simulink model "lunar_landing_modified"  (R2016b)
settings: Solver=ode5  StartTime=0.0  StopTime=100  FixedStep=0.01  RelTol=1e-3
undefined symbols (not defined in the file or in its folder): sigbuilder_block
settings Model: Creator=Thomas  LastModifiedBy=Thomas

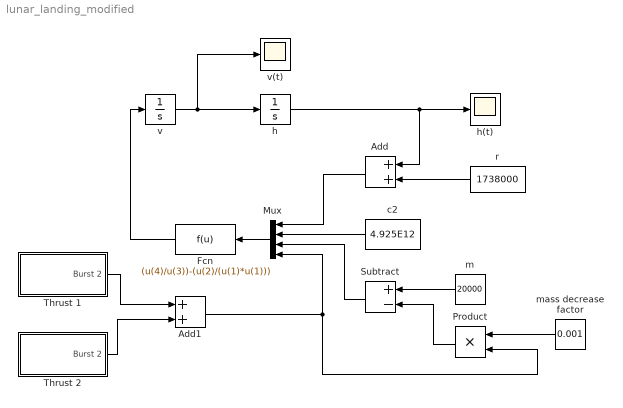
== system lunar_landing_modified ==
  Add : Sum
  Add1 : Sum
  Fcn : Fcn  Expr=(u(4)/u(3))-(u(2)/(u(1)*u(1)))
  Mux : Mux
  Product : Product
  Subtract : Sum  Inputs=+-
  Thrust 1 : Subsystem  Tag=STV Subsys  LoadFcn=sigbuilder_block('load',[448.5 411.75 550.5 334.5 ]);  StartFcn=sigbuilder_block('start');  StopFcn=sigbuilder_block('stop');  ClipboardFcn=sigbuilder_block('clipboard');  mask(Sigbuilder block){tuvar=[0:10]}
      mask help: Simulink:masks:SigbuilderBlock_MD
      mask init:
      | if ~strcmp(get_param(bdroot(gcbh),'SimulationStatus'),'stopped') tuvar = sigbuilder_block('maskInit'); end
      settings: CopyFcn=sigbuilder_block('copy');  DeleteFcn=sigbuilder_block('delete');  ModelCloseFcn=sigbuilder_block('modelClose');  PreSaveFcn=sigbuilder_block('preSave');  PauseFcn=sigbuilder_block('pause');  ContinueFcn=sigbuilder_block('continue');  NameChangeFcn=sigbuilder_block('namechange');  OpenFcn=sigbuilder_block('open',[446.25 33.75 550.5 334.5 ]);  CloseFcn=sigbuilder_block('close');
      mask Display: plot(0, 0, 100, 100,[2, 2, 32, 32, 2], [68, 8, 8, 68, 68],[32, 2], [38, 38], [32, 19, 2],[53, 60, 44], [32, 17, 17, 2],[16, 16, 31, 31]);txt = getActiveGroup(gcbh);text(2, 100, txt,'verticalAlignment', 'top');
  Thrust 2 : Subsystem  Tag=STV Subsys  LoadFcn=sigbuilder_block('load',[450.75 29.25 550.5 334.5 ]);  StartFcn=sigbuilder_block('start');  StopFcn=sigbuilder_block('stop');  ClipboardFcn=sigbuilder_block('clipboard');  mask(Sigbuilder block){tuvar=[0:10]}
      mask help: Simulink:masks:SigbuilderBlock_MD
      mask init:
      | if ~strcmp(get_param(bdroot(gcbh),'SimulationStatus'),'stopped') tuvar = sigbuilder_block('maskInit'); end
      settings: CopyFcn=sigbuilder_block('copy');  DeleteFcn=sigbuilder_block('delete');  ModelCloseFcn=sigbuilder_block('modelClose');  PreSaveFcn=sigbuilder_block('preSave');  PauseFcn=sigbuilder_block('pause');  ContinueFcn=sigbuilder_block('continue');  NameChangeFcn=sigbuilder_block('namechange');  OpenFcn=sigbuilder_block('open',[446.25 33.75 550.5 334.5 ]);  CloseFcn=sigbuilder_block('close');
      mask Display: plot(0, 0, 100, 100,[2, 2, 32, 32, 2], [68, 8, 8, 68, 68],[32, 2], [38, 38], [32, 19, 2],[53, 60, 44], [32, 17, 17, 2],[16, 16, 31, 31]);txt = getActiveGroup(gcbh);text(2, 100, txt,'verticalAlignment', 'top');
  c2 : Constant  Value=4.925E12
  h : Integrator  InitialCondition=1000
  h(t) : Scope
  m : Constant  Value=20000
  mass decrease factor : Constant  Value=0.001
  r : Constant  Value=1738000
  v : Integrator  InitialCondition=-10
  v(t) : Scope
  wires:
  v/1 -> h/1, v(t)/1
  Mux/1 -> Fcn/1
  h/1 -> h(t)/1, Add/1
  r/1 -> Add/2
  Add/1 -> Mux/1
  c2/1 -> Mux/2
  m/1 -> Subtract/1
  Thrust 2/1(Burst 2) -> Add1/2
  Add1/1 -> Product/2, Mux/4
  Fcn/1 -> v/1
  Thrust 1/1(Burst 2) -> Add1/1
  mass decrease factor/1 -> Product/1
  Product/1 -> Subtract/2
  Subtract/1 -> Mux/3

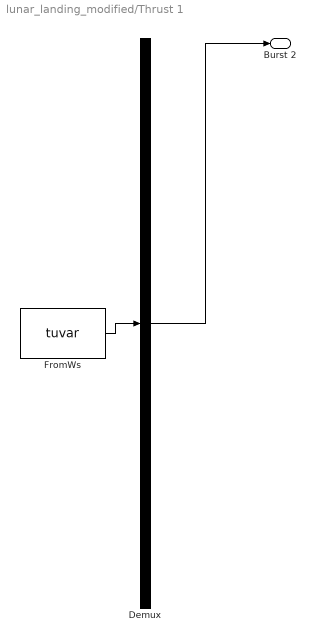
== system lunar_landing_modified/Thrust 1 ==
  Demux : Demux  Tag=STV Demux  Outputs=1
  FromWs : FromWorkspace  Tag=STV FromWs  VariableName=tuvar  SampleTime=0
      SigBuilderData=|
      | common.afterFinalStr = 'Extrapolate'
      | common.sampleTime = 0
      | dataSet.timeRange = [0 100]
      | dataSet.name = 'Group 1'
      | sbobj.Groups.Name = 'Group 1'
      | sbobj.Groups.Signals.Name = 'Burst 2'
      | sbobj.Groups.Signals.XData = [0 22 22 48.8 48.8 100]
      | sbobj.Groups.Signals.YData = [0 0 34000 34000 0 0]
      | sbobj.Groups.TimeRange = [0 100]
  Burst 2 : Outport  Tag=STV Outport
  wires:
  Demux/1 -> Burst 2/1
  FromWs/1 -> Demux/1

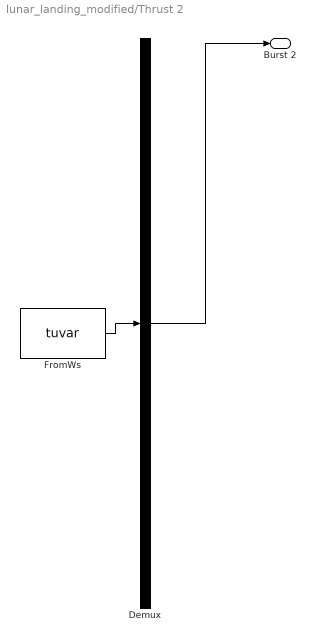
== system lunar_landing_modified/Thrust 2 ==
  Demux : Demux  Tag=STV Demux  Outputs=1
  FromWs : FromWorkspace  Tag=STV FromWs  VariableName=tuvar  SampleTime=0
      SigBuilderData=|
      | common.afterFinalStr = 'Extrapolate'
      | common.sampleTime = 0
      | dataSet.timeRange = [0 100]
      | dataSet.name = 'Group 1'
      | sbobj.Groups.Name = 'Group 1'
      | sbobj.Groups.Signals.Name = 'Burst 2'
      | sbobj.Groups.Signals.XData = [0 19.8 19.8 40.8 40.8 100]
      | sbobj.Groups.Signals.YData = [0 0 42000 42000 0 0]
      | sbobj.Groups.TimeRange = [0 100]
  Burst 2 : Outport  Tag=STV Outport
  wires:
  Demux/1 -> Burst 2/1
  FromWs/1 -> Demux/1
